simulink model "practice1"  (R2020b)
settings: Solver=VariableStepAuto  StartTime=0.0  StopTime=10.0  RelTol=1e-3
settings Model: Creator=yuto  LastModifiedBy=yuto

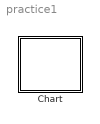
== system practice1 ==
  Chart : Stateflow chart  TreatAsAtomicUnit=on

== stateflow chart practice1/Chart ==
  state first
  state second
  state third
  state fourth
  (default) -> first
  second -> first [order 1] : [speed>10]
  third -> second [order 1] : [speed>30]
  third -> fourth [order 2] : [speed>50]
  first -> second : [speed<5]
  second -> third [order 2] : [speed<25]
  fourth -> third : [speed<40]
